simulink model "CACu"  (R2019a)
settings: Solver=VariableStepAuto  StartTime=0.0  StopTime=6  FixedStep=0.001  RelTol=1e-3
values from neighbouring files (symbols this model uses):
  B_EQ = 60    [CAC_ws.mat]    (also in CACu_ws.mat; abc_ws.mat)
  CURRENT_MAX = 3.14    [CAC_ws.mat]    (also in CACu_ws.mat; SimulationParameters.m = 3.14159265359; Simulation_ws.mat = 3.14159265359; TransferFunctions.m = 3.14159265359)
  damping_d = 1.6    [CAC_ws.mat]    (also in CACu_ws.mat = 0.9; abc_ws.mat = 0.770835010154; kalmanSSHumInput.m = 0.9; kalmanStateSpaceModellingHumInput.m = 0.9)
  epos_Ki = 1.19    [CAC_ws.mat]    (also in CACu_ws.mat; TransferFunctions.m; abc_ws.mat; kalmanSSHumInput.m)
  epos_Kp = 11.9    [CAC_ws.mat]    (also in CACu_ws.mat; TransferFunctions.m; abc_ws.mat; kalmanSSHumInput.m)
  f = [0.01 0.0100092155052 0.0100184395029 0.010027672001 0.0100369130073 0.0100461625297 0.0100554205759 0.010064687154 0.0100739622716 0.0100832459368 0.0100925381573 0.010101838941 ... (10000 elements, 1x10000)]    [abc_ws.mat]    (also in kalmanSSHumInput.m = logspace(-2,2,1e4); tests_analysis.m = (1/dt)*(0:(L/2))/L)
  GEAR_RATIO = 150    [CAC_ws.mat]    (also in CACu_ws.mat; abc_ws.mat)
  J_EQ = 0.47    [CAC_ws.mat]    (also in CACu_ws.mat; abc_ws.mat)
  Ki_adm = 0.18590515885    [CAC_ws.mat]    (also in CACu_ws.mat = 1.89921485516; abc_ws.mat = 1.89921485516)
  Kp_adm = 0.218227787186    [CAC_ws.mat]    (also in CACu_ws.mat = 0.277331265279; abc_ws.mat = 0.277331265279)
  Ksea = 104    [CAC_ws.mat]    (also in CACu_ws.mat; abc_ws.mat)
  stiffness_d = 1.04    [CAC_ws.mat]    (also in CACu_ws.mat = 3.874; abc_ws.mat = 14.0803237251; kalmanSSHumInput.m = 3.874; kalmanStateSpaceModellingHumInput.m = 3.874)
  Threaded_Ts = 0.001    [CAC_ws.mat]    (also in CACu_ws.mat; SimulationParameters.m; Simulation_ws.mat; abc_ws.mat)
  TORQUE_CONST = 0.0603    [CAC_ws.mat]    (also in CACu_ws.mat; abc_ws.mat)
undefined symbols (not defined in the file or in its folder): DiscIntNeverNeededParam
libraries: simulink x2, instrumentlib x2, discretizing x1
Description:
  | Collocated Admittance Control study for the acceleration-based SEA Transparency Control
settings Model: OrderedModelArguments=off  Creator=Leonardo Felipe  LastModifiedBy=Leonardo Felipe
settings DataIOCC: LimitDataPoints=on  MaxDataPoints=23000  SignalLogging=off  ReturnWorkspaceOutputs=off

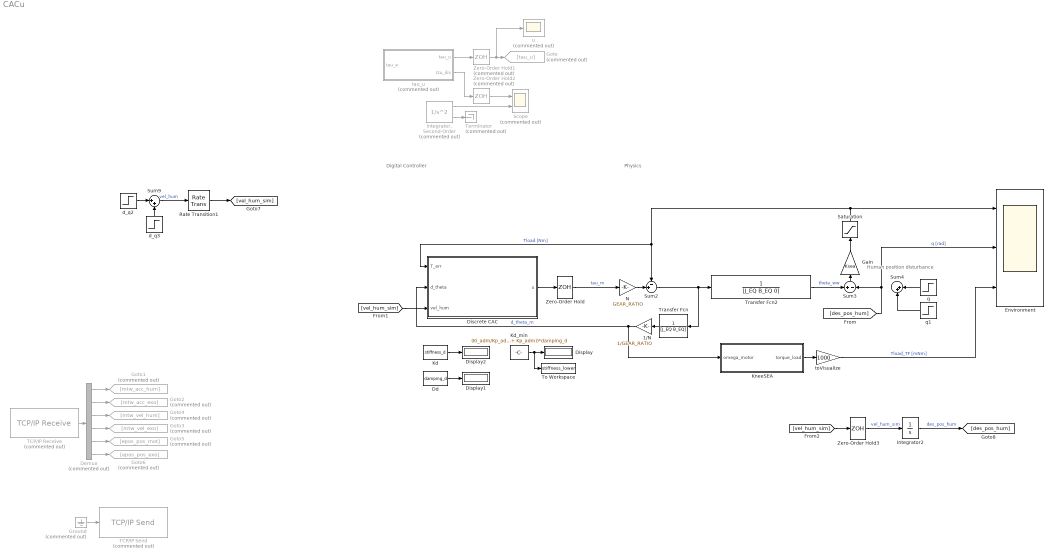
== system CACu ==
  note: Digital Controller
  note: Human position disturbance
  note: Physics
  1/N : Gain  Gain=1/GEAR_RATIO
  Dd : Constant  Value=damping_d
  Demux : Demux  Commented=on  Outputs=6
  Discrete CAC : Subsystem  TreatAsAtomicUnit=on  SystemSampleTime=Threaded_Ts
  Display : Display
      settings: Decimation=5
  Display1 : Display
      settings: Decimation=5
  Display2 : Display
      settings: Decimation=5
  Environment : Scope  NumInputPorts=3
  Gain : Gain  Gain=Ksea
  Goto : Goto  Commented=on  GotoTag=tau_u
  Goto1 : Goto  Commented=on  GotoTag=mtw_acc_hum
  Goto2 : Goto  Commented=on  GotoTag=mtw_acc_exo
  Goto3 : Goto  Commented=on  GotoTag=mtw_vel_exo
  Goto4 : Goto  Commented=on  GotoTag=mtw_vel_hum
  Goto5 : Goto  Commented=on  GotoTag=epos_pos_mot
  Goto6 : Goto  Commented=on  GotoTag=epos_pos_exo
  Ground : Ground  Commented=on
  "Integrator, Second-Order" : SecondOrderIntegrator  Commented=on
  Integrator2 : Integrator
  Kd : Constant  Value=stiffness_d
  Kd_min : Constant  Value=(Ki_adm/Kp_adm - 1/J_EQ*(damping_d/(1 - stiffness_d/Ksea) + Kp_adm))*damping_d
  KneeSEA : Subsystem
  N : Gain  Gain=GEAR_RATIO
  Rate Transition1 : RateTransition  OutPortSampleTime=Threaded_Ts
  Saturation : Saturate  UpperLimit=250  LowerLimit=-250
  Scope : Scope  Commented=on  NumInputPorts=2
  Sum2 : Sum  Inputs=-+|
  Sum3 : Sum  Inputs=+-
  Sum4 : Sum  Inputs=|++
  Sum9 : Sum  Inputs=|++
  TCP/IP Receive : instrumentlib/TCP//IP Receive  Commented=on  Host=127.0.0.1  Port=23000  DataSize="[1  6]"  EnableBlockingMode=on  Timeout=0.3  SampleTime=Threaded_Ts  DataType=single  ByteOrder=BigEndian  ASCIIFormatting=%f,  Terminator=LF
      settings: SourceProductName=Instrument Control Toolbox
  TCP/IP Send : instrumentlib/TCP//IP Send  Commented=on  Host=127.0.0.1  Port=23001  EnableBlockingMode=on  Timeout=0.3  ByteOrder=BigEndian  TransferDelay=off
      settings: SourceProductName=Instrument Control Toolbox
  Terminator : Terminator  Commented=on
  To Workspace : ToWorkspace  VariableName=stiffness_lower  SampleTime=-1
      settings: MaxDataPoints=1
  Transfer Fcn : TransferFcn  Denominator=[J_EQ B_EQ]
  Transfer Fcn2 : TransferFcn  Denominator=[J_EQ B_EQ 0]
  Zero-Order Hold : ZeroOrderHold  SampleTime=Threaded_Ts
  Zero-Order Hold1 : ZeroOrderHold  Commented=on  SampleTime=Threaded_Ts
  Zero-Order Hold2 : ZeroOrderHold  Commented=on  SampleTime=Threaded_Ts
  Zero-Order Hold3 : ZeroOrderHold  SampleTime=Threaded_Ts
  d_q2 : Step  SampleTime=0.008
  d_q3 : Step  Time=1.4  After=-1  SampleTime=0.008
  q : Step  SampleTime=0
  q1 : Step  Time=1.4  After=-1  SampleTime=0
  tau_u : Subsystem  Commented=on  TreatAsAtomicUnit=on  SystemSampleTime=Threaded_Ts
  toVisualize : Gain  Gain=1000
  u : Scope  Commented=on
  wires:
  Sum2/1 -> Transfer Fcn2/1, Transfer Fcn/1
  Transfer Fcn/1 -> 1/N/1
  Sum3/1 -> Gain/1
  Gain/1 -> Saturation/1
  Zero-Order Hold1/1 -> u/1, Goto/1
  tau_u/1(tau_u) -> Zero-Order Hold1/1
  q/1 -> Sum4/1
  q1/1 -> Sum4/2
  Saturation/1 -> Environment/1, Sum2/1, Discrete CAC/1(T_err)  "Tload [Nm]"
  [des_pos_hum] -> Sum3/2, Environment/2  "q [rad]"
  d_q3/1 -> Sum9/2
  d_q2/1 -> Sum9/1
  Rate Transition1/1 -> [vel_hum_sim]
  Sum9/1 -> Rate Transition1/1  "vel_hum"
  "Integrator, Second-Order"/2 -> Terminator/1
  "Integrator, Second-Order"/1 -> Scope/2
  tau_u/2(I2u_dis) -> Zero-Order Hold2/1
  Zero-Order Hold2/1 -> Scope/1
  TCP/IP Receive/1 -> Demux/1
  Demux/1 -> Goto1/1
  Demux/2 -> Goto2/1
  Demux/3 -> Goto4/1
  Demux/4 -> Goto3/1
  Demux/5 -> Goto5/1
  Demux/6 -> Goto6/1
  Ground/1 -> TCP/IP Send/1
  [vel_hum_sim] -> Zero-Order Hold3/1
  Integrator2/1 -> [des_pos_hum]  "des_pos_hum"
  Discrete CAC/1(u) -> Zero-Order Hold/1
  Zero-Order Hold/1 -> N/1  "tau_m"
  N/1 -> Sum2/2
  1/N/1 -> KneeSEA/1(omega_motor), Discrete CAC/2(d_theta)  "d_theta_m"
  Transfer Fcn2/1 -> Sum3/1  "theta_ww"
  KneeSEA/1(torque_load) -> toVisualize/1
  toVisualize/1 -> Environment/3  "Tload_TF [mNm]"
  Dd/1 -> Display1/1
  Kd/1 -> Display2/1
  [vel_hum_sim] -> Discrete CAC/3(vel_hum)
  Zero-Order Hold3/1 -> Integrator2/1  "vel_hum_sim"
  Kd_min/1 -> To Workspace/1, Display/1

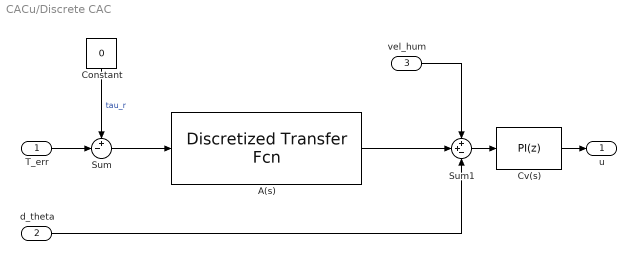
== system CACu/Discrete CAC ==
  T_err : Inport  SampleTime=Threaded_Ts
  d_theta : Inport  Port=2  SampleTime=Threaded_Ts
  vel_hum : Inport  Port=3  SampleTime=Threaded_Ts
  A(s) : discretizing/Discretized Transfer Fcn  Numerator=[(1 - stiffness_d/Ksea) 0]  Denominator=[damping_d stiffness_d]  AbsTol=auto  SampleTime=Threaded_Ts  method=zoh  Wc=1
      settings: SourceProductName=Simulink  SourceProductBaseCode=SL
  Constant : Constant  Value=0  SampleTime=Threaded_Ts
  Cv(s) : simulink/Continuous/PID Controller  Controller=PI  Form=Parallel  TimeDomain=Discrete-time  SampleTime=Threaded_Ts  IntegratorMethod=Forward Euler  FilterMethod=Forward Euler  ControllerParametersSource=internal  P=Kp_adm  I=Ki_adm  D=0  UseFilter=on  N=100  TunerSelectOption=Transfer Function Based (PID Tuner App)  InitialConditionSource=internal  InitialConditionForIntegrator=0  InitialConditionForFilter=0  DifferentiatorICPrevScaledInput=0  ExternalReset=none  TrackingMode=off  Kt=1  LimitOutput=off  UpperSaturationLimit=inf  LowerSaturationLimit=-inf  LinearizeAsGain=on  AntiWindupMode=none  Kb=1  POutMin=[]  POutMax=[]  IOutMin=[]  IOutMax=[]  DOutMin=[]  DOutMax=[]  NOutMin=[]  NOutMax=[]  SumOutMin=[]  SumOutMax=[]  SaturationOutMin=[]  SaturationOutMax=[]  PParamMin=[]  PParamMax=[]  IParamMin=[]  IParamMax=[]  DParamMin=[]  DParamMax=[]  NParamMin=[]  NParamMax=[]  KbParamMin=[]  KbParamMax=[]  KtParamMin=[]  KtParamMax=[]  KbOutMin=[]  KbOutMax=[]  KtOutMin=[]  KtOutMax=[]  IntegratorOutMin=[]  IntegratorOutMax=[]  FilterOutMin=[]  FilterOutMax=[]  SumI1OutMin=[]  SumI1OutMax=[]  SumI2OutMin=[]  SumI2OutMax=[]  SumI3OutMin=[]  SumI3OutMax=[]  SumI4OutMin=[]  SumI4OutMax=[]  SumDOutMin=[]  SumDOutMax=[]  DifferentiatorOutMin=[]  DifferentiatorOutMax=[]  FilterDiffOutCoefMin=[]  FilterDiffOutCoefMax=[]  ReciprocalOutMin=[]  ReciprocalOutMax=[]  SumDenOutMin=[]  SumDenOutMax=[]  SumNumOutMin=[]  SumNumOutMax=[]  DivideOutMin=[]  DivideOutMax=[]  IntegratorContinuousStateAttributes=''  IntegratorStateMustResolveToSignalObject=off  IntegratorRTWStateStorageClass=Auto  FilterContinuousStateAttributes=''  FilterStateMustResolveToSignalObject=off  FilterRTWStateStorageClass=Auto  ParallelPVariant=InternalParameters  IdealPVariant=Disabled  IVariant=InternalParameters  DVariant=Disabled  IntegratorVariant=Discrete  SatVariant=Disabled  AWVariant=Passthrough  PCopyVariant=Disabled  TRVariant=Disabled  FdbkBlocksVariant=Forward  IdealPFdbkVariant=Disabled  SatFdbkVariant=Disabled  DerivativeFilterVariant=Disabled  NVariant=Disabled  NCopyVariant=Disabled_SignalSpec  FilterICVariant=Disabled  IntegratorICVariant=InternalICs  ExternalResetVariant=Disabled  TRSumVariant=Passthrough  SumFdbkVariant=Disabled  SumVariant=Sum_PI
  Sum : Sum  Inputs=+-|
  Sum1 : Sum  Inputs=++-
  u : Outport
  wires:
  d_theta/1 -> Sum1/3
  T_err/1 -> Sum/2
  Sum/1 -> A(s)/1
  Constant/1 -> Sum/1  "tau_r"
  Sum1/1 -> Cv(s)/1
  vel_hum/1 -> Sum1/1
  Cv(s)/1 -> u/1
  A(s)/1 -> Sum1/2

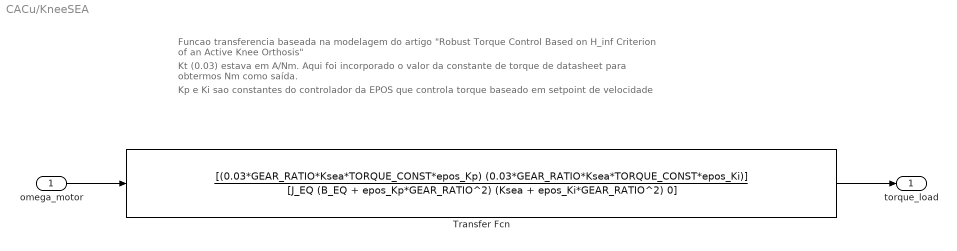
== system CACu/KneeSEA ==
  note: Kp e Ki sao constantes do controlador da EPOS que controla torque baseado em setpoint de velocidade
  note: Kt (0.03) estava em A/Nm. Aqui foi incorporado o valor da constante de torque de datasheet para obtermos Nm como saída.
  note: Funcao transferencia baseada na modelagem do artigo "Robust Torque Control Based on H_inf Criterion of an Active Knee Orthosis"
  omega_motor : Inport  OutDataTypeStr=double  Unit=rad/s  PortDimensions=1
  Transfer Fcn : TransferFcn  Numerator=[(0.03*GEAR_RATIO*Ksea*TORQUE_CONST*epos_Kp) (0.03*GEAR_RATIO*Ksea*TORQUE_CONST*epos_Ki)]  Denominator=[J_EQ (B_EQ + epos_Kp*GEAR_RATIO^2) (Ksea + epos_Ki*GEAR_RATIO^2) 0]
  torque_load : Outport  OutDataTypeStr=double  Unit=N*m  PortDimensions=1
  wires:
  omega_motor/1 -> Transfer Fcn/1
  Transfer Fcn/1 -> torque_load/1

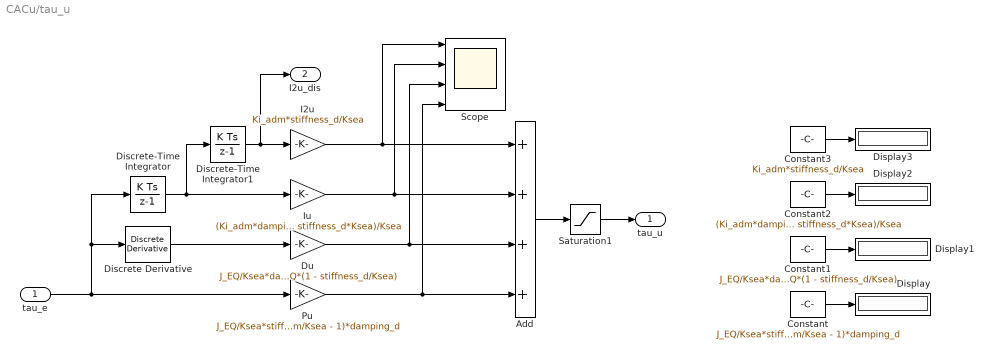
== system CACu/tau_u ==
  tau_e : Inport  SampleTime=0.001
  Add : Sum  Inputs=++++
  Constant : Constant  Value=J_EQ/Ksea*stiffness_d + (Kp_adm/Ksea - 1)*damping_d  SampleTime=0.001
  Constant1 : Constant  Value=J_EQ/Ksea*damping_d - J_EQ*(1 - stiffness_d/Ksea)  SampleTime=0.001
  Constant2 : Constant  Value=(Ki_adm*damping_d + Kp_adm*stiffness_d - stiffness_d*Ksea)/Ksea  SampleTime=0.001
  Constant3 : Constant  Value=Ki_adm*stiffness_d/Ksea  SampleTime=0.001
  Discrete Derivative : simulink/Discrete/Discrete Derivative  gainval=1.0  ICPrevScaledInput=0.0  OutMin=[]  OutMax=[]  OutDataType=fixdt(1, 16)  OutScaling=2^-10  DoSatur=off
  Discrete-Time Integrator : DiscreteIntegrator  SampleTime=0.001  ICPrevOutput=DiscIntNeverNeededParam  ICPrevScaledInput=DiscIntNeverNeededParam
  Discrete-Time Integrator1 : DiscreteIntegrator  SampleTime=0.001  ICPrevOutput=DiscIntNeverNeededParam  ICPrevScaledInput=DiscIntNeverNeededParam
  Display{,1..3} (4 alike) : Display
      settings: Decimation=5
  Du : Gain  Gain=J_EQ/Ksea*damping_d - J_EQ*(1 - stiffness_d/Ksea)
  I2u : Gain  Gain=Ki_adm*stiffness_d/Ksea
  Iu : Gain  Gain=(Ki_adm*damping_d + Kp_adm*stiffness_d - stiffness_d*Ksea)/Ksea
  Pu : Gain  Gain=J_EQ/Ksea*stiffness_d + (Kp_adm/Ksea - 1)*damping_d
  Saturation1 : Saturate  UpperLimit=TORQUE_CONST*CURRENT_MAX  LowerLimit=-TORQUE_CONST*CURRENT_MAX
  Scope : Scope  NumInputPorts=4
  tau_u : Outport  SampleTime=0.001
  I2u_dis : Outport  Port=2
  wires:
  Add/1 -> Saturation1/1
  Du/1 -> Scope/3, Add/3
  Discrete Derivative/1 -> Du/1
  Iu/1 -> Scope/2, Add/2
  Pu/1 -> Scope/4, Add/4
  Discrete-Time Integrator/1 -> Discrete-Time Integrator1/1, Iu/1
  I2u/1 -> Scope/1, Add/1
  Discrete-Time Integrator1/1 -> I2u_dis/1, I2u/1
  tau_e/1 -> Pu/1, Discrete-Time Integrator/1, Discrete Derivative/1
  Saturation1/1 -> tau_u/1
  Constant/1 -> Display/1
  Constant1/1 -> Display1/1
  Constant2/1 -> Display2/1
  Constant3/1 -> Display3/1
